simulink model "trabalhofinal_vR2012a"  (R2012a)
settings: Solver=FixedStepDiscrete  StartTime=0.0  StopTime=0.5  FixedStep=0.1e-6  MaxStep=50e-6
undefined symbols (not defined in the file): DiscIntNeverNeededParam, Ipac0, Vpac0
libraries: powerlib x36, simulink x19, fuzblock x7, powerlib_extras x2, powerlib_meascontrol x2
(part 1 of 3)
settings Model: Creator=Arthur  LastModifiedBy=Thainan
settings DataIOCC: FinalStateName=SimState  InitialState=SimState  LimitDataPoints=on  SaveCompleteFinalSimState=on  SaveFormat=Array  SignalLoggingSaveFormat=ModelDataLogs  SaveOutput=off  SignalLogging=off  DSMLogging=off  SaveTime=off  ReturnWorkspaceOutputs=off  ReturnWorkspaceOutputsName=States
settings OptimizationCC: ExpressionDepthLimit=2147483647  LifeSpan=inf  SimCompilerOptimization=Off
settings DebuggingCC: UnderspecifiedInitializationDetection=Classic  MergeDetectMultiDrivingBlocksExec=none  SolverPrmCheckMsg=warning  FcnCallInpInsideContextMsg=Enable All  StateNameClashWarn=warning  SFUnexpectedBacktrackingDiag=warning  SFNoUnconditionalDefaultTransitionDiag=warning
settings HardwareCC: ProdBitPerPointer=32  ProdLargestAtomicFloat=None  ProdIntDivRoundTo=Undefined  ProdEndianess=Unspecified  ProdWordSize=32  ProdHWDeviceType=32-bit Generic
settings ModelReferenceCC: PropagateSignalLabelsOutOfModel=off
settings SFSimCC: SimUseLocalCustomCode=off
settings RTWCC: RTWUseLocalCustomCode=off  RTWCompilerOptimization=Off
settings GRTTargetCC: CodeReplacementLibrary=C89/C90 (ANSI)  GeneratePreprocessorConditionals=Disable all  CPPClassGenCompliant=off

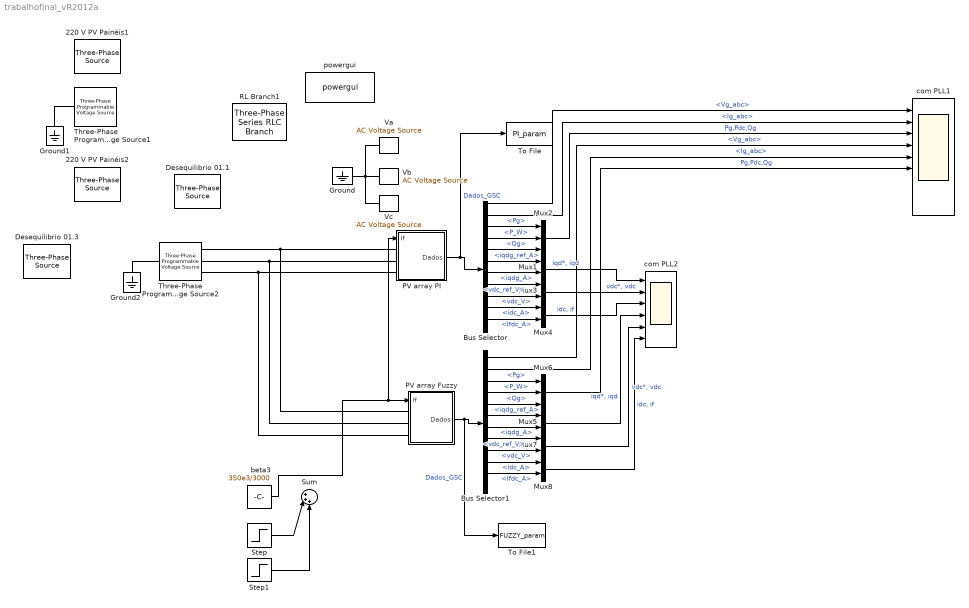
== system trabalhofinal_vR2012a ==
  220 V PV Painéis1 : powerlib/Electrical Sources/Three-Phase Source  InternalConnection=Yg  VoltagePhases=on  Voltage=120e3  PhaseAngle=0  Voltage_phases=[ 1.04183 1.09667 1.03168]*127.017  PhaseAngles_phases=[ -0.131766 -117.596 121.449]  Frequency=60  NonIdealSource=off  SpecifyImpedance=on  Resistance=0.8929  Inductance=16.58e-3  ShortCircuitLevel=100e6  BaseVoltage=120e3  XRratio=10  BusType=swing  Pref=0  Qref=0  Prefabc=[1 1 1]*400e3  Qrefabc=[1 1 1]*100  Qmin=[-1 -1 -1]*(-inf)  Qmax=[1 1 1]*inf
  220 V PV Painéis2 : powerlib/Electrical Sources/Three-Phase Source  InternalConnection=Yg  VoltagePhases=on  Voltage=120e3  PhaseAngle=0  Voltage_phases=[1 1 1]*127  PhaseAngles_phases=[ 0 -120 120]  Frequency=60  NonIdealSource=off  SpecifyImpedance=on  Resistance=0.8929  Inductance=16.58e-3  ShortCircuitLevel=100e6  BaseVoltage=120e3  XRratio=10  BusType=PQ  Pref=0  Qref=0  Prefabc=[1 1 1]*400e3  Qrefabc=[1 1 1]*100  Qmin=[-1 -1 -1]*(-inf)  Qmax=[1 1 1]*inf
  Bus Selector : BusSelector  OutputSignals=Dados_grid.Vg_abc,Dados_grid.Ig_abc,Dados_grid.Pg,DadosCC.P_W,Dados_grid.Qg,DadosCtrlCorr.iqdg_ref_A,DadosCtrlCorr.iqdg_A,DadosCtrlTensao.vdc_ref_V,DadosCtrlTensao.vdc_V,DadosCC.idc_A,DadosCC.Ifdc_A,DadosPLL.rog_rad
  Bus Selector1 : BusSelector  OutputSignals=Dados_grid.Vg_abc,Dados_grid.Ig_abc,Dados_grid.Pg,DadosCC.P_W,Dados_grid.Qg,DadosCtrlCorr.iqdg_ref_A,DadosCtrlCorr.iqdg_A,DadosCtrlTensao.vdc_ref_V,DadosCtrlTensao.vdc_V,DadosCC.idc_A,DadosCC.Ifdc_A,DadosPLL.rog_rad
  Desequilibrio 01.1 : powerlib/Electrical Sources/Three-Phase Source  InternalConnection=Yg  VoltagePhases=on  Voltage=120e3  PhaseAngle=0  Voltage_phases=[ 1.2 1 0.80]*127  PhaseAngles_phases=[ 0 -125 115]  Frequency=60  NonIdealSource=off  SpecifyImpedance=on  Resistance=0.8929  Inductance=16.58e-3  ShortCircuitLevel=100e6  BaseVoltage=120e3  XRratio=10  BusType=PQ  Pref=0  Qref=0  Prefabc=[1 1 1]*400e3  Qrefabc=[1 1 1]*100  Qmin=[-1 -1 -1]*(-inf)  Qmax=[1 1 1]*inf
  Desequilibrio 01.3 : powerlib/Electrical Sources/Three-Phase Source  InternalConnection=Yg  VoltagePhases=on  Voltage=120e3  PhaseAngle=0  Voltage_phases=[1 1 1]*440/sqrt(3)  PhaseAngles_phases=[ 0 -120 120]-90  Frequency=60  NonIdealSource=off  SpecifyImpedance=on  Resistance=0.8929  Inductance=16.58e-3  ShortCircuitLevel=100e6  BaseVoltage=120e3  XRratio=10  BusType=PQ  Pref=0  Qref=0  Prefabc=[1 1 1]*400e3  Qrefabc=[1 1 1]*100  Qmin=[-1 -1 -1]*(-inf)  Qmax=[1 1 1]*inf
  Ground : powerlib/Elements/Ground  LConnTagsString=a
  Ground1 : powerlib/Elements/Ground  LConnTagsString=a
  Ground2 : powerlib/Elements/Ground  LConnTagsString=a
  Mux{1,3..5,7..8} (6 alike) : Mux  Inputs=2
  Mux2 : Mux  Inputs=3
  Mux6 : Mux  Inputs=3
  PV array Fuzzy : Subsystem  mask(Usina Fotovoltáica){nom=[450e3 440 60], S0_pu=(350e3 +1j*0)/450e3, V0_pu=1+0*1j, C_DClink=2*4700e-6, Vdc_nom=3000, filtro_RL_pu=[0.03 0.3], GSC_PLL=[2*pi*100 sqrt(2) 2*pi*60], GSC_Ci_Ti=1e-3, GSC_Cv=[sqrt(2)  0.01*(1/1e-3)*2*pi], PWM_freq_grid=10e3, Ts_control=100e-6}
      mask prompts: nom "[Pn (VA), Vn (Vrms), fn (Hz)]:"; S0_pu "Potência aparente inicial (complexo), S0 [pu]"; V0_pu "Tensão inicial na barra (complexo), V0 [pu]"; C_DClink "C_DClink (F):"; Vdc_nom "V_DClink (V):"; filtro_RL_pu "Filtro RL [Rg_pu Lg_pu]"; GSC_PLL "Parâmetros PLL [wc qsi wff]"; GSC_Ci_Ti "Constante de tempo - Compensador de corrente GSC_Ci_Ti (s)"; GSC_Cv "Parametros controlador de tensão GSC [Cv_qsi Cv_wn]"; PWM_freq_grid "Frequencia de chaveamento do GSC"; Ts_control "Ts do controle"
      mask help: Usina fotovoltáica com inicialização.
      mask init:
      | fuzzyControl = readfis('fuzzyControl');
      | 
      | %Aquisição de dados
      | 
      | Sb = nom(1);
      | Vb = nom(2)/sqrt(3);
      | fb = nom(3); wb = 2*pi*fb;
      | S0_pu = S0_pu;
      | V0_pu = V0_pu;
      | 
      | C_DClink = C_DClink;
      | Vdc_nom = Vdc_nom;
      | 
      | Rg_pu = filtro_RL_pu(1);
      | Lg_pu = filtro_RL_pu(2);
      | 
      | GSC_PLL_wc = GSC_PLL(1);
      | GSC_PLL_qsi = GSC_PLL(2);
      | GSC_PLL_wff = GSC_PLL(3);
      | 
      | GSC_Ci_Ti = GSC_Ci_Ti;
      | 
      | GSC_Cv_qsi = GSC_Cv(1);
      | GSC_Cv_wn = GSC_Cv(2);
      | 
      | PWM_freq_grid = PWM_freq_grid;
      | 
      | Ib = Sb/(3*Vb);         % A
      | Zb = Vb/Ib;             % ohm
      | Lb = Zb/(2*pi*fb);      % Hz
      | wb = 2*pi*fb;           % rad/s
      | Yb = Vb/wb;             % wb
      | 
      | %% Condições iniciais
      | P0 = Sb*real(S0_pu);
      | Q0 = Sb*imag(S0_pu);
      | 
      | %% Controle GSC
      | % Projeto Controle de Corrente
      | Rg = Rg_pu*Zb;
      | Lg = Lg_pu*Lb;
      | 
      | GSC_Ci_kp = Lg/GSC_Ci_Ti;
      | GSC_Ci_ki = Rg/GSC_Ci_Ti;
      | 
      | %% Controle do Link DC
      | GSC_Cv_kv = -(3/2)*Vb*sqrt(2)/(Vdc_nom*C_DClink);
      | % Livro
      | 
      | GSC_Cv_kp = abs(2*GSC_Cv_qsi*GSC_Cv_wn/GSC_Cv_kv);
      | GSC_Cv_ki = abs((GSC_Cv_wn^2)/GSC_Cv_kv);
      | % Fontes Alternativas
      | % GSC_Cv_kp = 2*GSC_Cv_qsi*C_DClink*GSC_Cv_wn;
      | % GSC_Cv_ki = C_DClink*GSC_Cv_wn^2;
      | % 
      | % GSC_Cv_kp = 2.4806;
      | % GSC_Cv_ki = 667.9748;
      | 
      | %% Inicialização do Controle
      | Vgq_e = Vb*abs(V0_pu)*sqrt(2);
      | Vgd_e = 0; % PLL responsável
      | 
      | Igd_e = (2/3)*Q0/Vgq_e;
      | Igq_e = (2/3)*P0/Vgq_e;
      | 
      | GSC_Uq_e = Rg*Igq_e;
      | GSC_Ud_e = Rg*Igd_e;
      | 
      | %% Inicialização da fonte de corrente
      | If0 = P0/Vdc_nom;
      | 
      | % %% Incerteza nos parâmteros
      | % Rg = 0.8*Rg_pu*Zb;
      | % Lg = 0.8*Lg_pu*Lb;
      mask Help:
      | Dicas
      | Parâmtros da malha de corrente:
      | 	tau_i: constante de tempo de corrente 0.5 a 3ms;
      | 
      | Parâmetros do controlador de tensão
      | 	qsi_i: amortecimento critico, sqrt(2);
      | 	wn: frequência de oscilação natural.
      | 	Deve ser menor que a frequencia da malha de corrente, assim wn = 0.1*(2*pi/tau_i)]
      | 
      | Frequência de chaveamento
      | 	O valor ótimo é 10e3 Hz
      | 
      | Ts o controle
      | 	O controle pode ser feito em uma taxa de amostragem diferente da simulação do sistema, mas deve ser levado em condideração a frequência de chaveamento.
  PV array PI : Subsystem  mask(Usina Fotovoltáica){nom=[450e3 440 60], S0_pu=(350e3 +1j*0)/450e3, V0_pu=1+0*1j, C_DClink=2*4700e-6, Vdc_nom=3000, filtro_RL_pu=[0.03 0.3], GSC_PLL=[2*pi*100 sqrt(2) 2*pi*60], GSC_Ci_Ti=1e-3, GSC_Cv=[sqrt(2)  0.01*(1/1e-3)*2*pi], PWM_freq_grid=10e3, Ts_control=100e-6}
      mask prompts: nom "[Pn (VA), Vn (Vrms), fn (Hz)]:"; S0_pu "Potência aparente inicial (complexo), S0 [pu]"; V0_pu "Tensão inicial na barra (complexo), V0 [pu]"; C_DClink "C_DClink (F):"; Vdc_nom "V_DClink (V):"; filtro_RL_pu "Filtro RL [Rg_pu Lg_pu]"; GSC_PLL "Parâmetros PLL [wc qsi wff]"; GSC_Ci_Ti "Constante de tempo - Compensador de corrente GSC_Ci_Ti (s)"; GSC_Cv "Parametros controlador de tensão GSC [Cv_qsi Cv_wn]"; PWM_freq_grid "Frequencia de chaveamento do GSC"; Ts_control "Ts do controle"
      mask help: Usina fotovoltáica com inicialização.
      mask init:
      | %Aquisição de dados
      | 
      | Sb = nom(1);
      | Vb = nom(2)/sqrt(3);
      | fb = nom(3); wb = 2*pi*fb;
      | S0_pu = S0_pu;
      | V0_pu = V0_pu;
      | 
      | C_DClink = C_DClink;
      | Vdc_nom = Vdc_nom;
      | 
      | Rg_pu = filtro_RL_pu(1);
      | Lg_pu = filtro_RL_pu(2);
      | 
      | GSC_PLL_wc = GSC_PLL(1);
      | GSC_PLL_qsi = GSC_PLL(2);
      | GSC_PLL_wff = GSC_PLL(3);
      | 
      | GSC_Ci_Ti = GSC_Ci_Ti;
      | 
      | GSC_Cv_qsi = GSC_Cv(1);
      | GSC_Cv_wn = GSC_Cv(2);
      | 
      | PWM_freq_grid = PWM_freq_grid;
      | 
      | Ib = Sb/(3*Vb);         % A
      | Zb = Vb/Ib;             % ohm
      | Lb = Zb/(2*pi*fb);      % Hz
      | wb = 2*pi*fb;           % rad/s
      | Yb = Vb/wb;             % wb
      | 
      | %% Condições iniciais
      | P0 = Sb*real(S0_pu);
      | Q0 = Sb*imag(S0_pu);
      | 
      | %% Controle GSC
      | % Projeto Controle de Corrente
      | Rg = Rg_pu*Zb;
      | Lg = Lg_pu*Lb;
      | 
      | GSC_Ci_kp = (Lg)/GSC_Ci_Ti;
      | GSC_Ci_ki = (Rg)/GSC_Ci_Ti;
      | 
      | %% Controle do Link DC
      | GSC_Cv_kv = -(3/2)*Vb*sqrt(2)/(Vdc_nom*C_DClink);
      | % Livro
      | 
      | GSC_Cv_kp = abs(2*GSC_Cv_qsi*GSC_Cv_wn/GSC_Cv_kv);
      | GSC_Cv_ki = abs((GSC_Cv_wn^2)/GSC_Cv_kv);
      | % Fontes Alternativas
      | % GSC_Cv_kp = 2*GSC_Cv_qsi*C_DClink*GSC_Cv_wn;
      | % GSC_Cv_ki = C_DClink*GSC_Cv_wn^2;
      | % 
      | % GSC_Cv_kp = 2.4806;
      | % GSC_Cv_ki = 667.9748;
      | 
      | %% Inicialização do Controle
      | Vgq_e = Vb*abs(V0_pu)*sqrt(2);
      | Vgd_e = 0; % PLL responsável
      | 
      | Igd_e = (2/3)*Q0/Vgq_e;
      | Igq_e = (2/3)*P0/Vgq_e;
      | 
      | GSC_Uq_e = Rg*Igq_e;
      | GSC_Ud_e = Rg*Igd_e;
      | 
      | %% Inicialização da fonte de corrente
      | If0 = P0/Vdc_nom;
      | 
      | % %% Incerteza nos parâmteros
      | % Rg = 0.8*Rg_pu*Zb;
      | % Lg = 0.8*Lg_pu*Lb;
      mask Help:
      | Dicas
      | Parâmtros da malha de corrente:
      | 	tau_i: constante de tempo de corrente 0.5 a 3ms;
      | 
      | Parâmetros do controlador de tensão
      | 	qsi_i: amortecimento critico, sqrt(2);
      | 	wn: frequência de oscilação natural.
      | 	Deve ser menor que a frequencia da malha de corrente, assim wn = 0.1*(2*pi/tau_i)]
      | 
      | Frequência de chaveamento
      | 	O valor ótimo é 10e3 Hz
      | 
      | Ts o controle
      | 	O controle pode ser feito em uma taxa de amostragem diferente da simulação do sistema, mas deve ser levado em condideração a frequência de chaveamento.
  RL Branch1 : powerlib/Elements/Three-Phase Series RLC Branch  LConnTagsString=A|B|C  RConnTagsString=A|B|C  BranchType=RL  Resistance=0.001  Inductance=0.3e-3  Capacitance=1e-6  Measurements=None
  Step : Step  Time=0.1  After=-0.2*350e3/3000
  Step1 : Step  Time=0.25  After=0.4*350e3/3000
  Sum : Sum  Inputs=|+++
  Three-Phase Programmable Voltage Source1 : powerlib/Electrical Sources/Three-Phase Programmable Voltage Source  PositiveSequence=[220 0 60]  VariationEntity=None  VariationType=Table of time-amplitude pairs  VariationTypeAlt=Step  VariationStep=0.5  VariationRate=10  VariationMagnitude=0.3  VariationFrequency=2  VariationTiming=[1 2]  VariationPhaseA=off  Amplitudes=[1 0.5 0.5 0.5]  TimeValues=[0 0.2 0.2+5*(1/60) 2.5]  HarmonicGeneration=on  HarmonicA=[3 0.1 -25 1]  HarmonicB=[2 0.1 35 2]  Timing="[0.03  0.1]"  BusType=swing  Pref=0  Qref=0  Qmin=-inf  Qmax=inf
  Three-Phase Programmable Voltage Source2 : powerlib/Electrical Sources/Three-Phase Programmable Voltage Source  PositiveSequence=[440 -90 60]  VariationEntity=None  VariationType=Table of time-amplitude pairs  VariationTypeAlt=Step  VariationStep=0.5  VariationRate=10  VariationMagnitude=0.3  VariationFrequency=2  VariationTiming=[0.1 0.3]  VariationPhaseA=off  Amplitudes=[1 0.5 1 1]  TimeValues=[0 0.1 0.3 2.5]  HarmonicGeneration=on  HarmonicA=[3 0.1 -25 0]  HarmonicB=[2 0.2 35 2]  Timing="[0.15  0.25]"  BusType=swing  Pref=0  Qref=0  Qmin=-inf  Qmax=inf
  To File : ToFile  Filename=PI_param  MatrixName=PI  SaveFormat=Timeseries
  To File1 : ToFile  Filename=FUZZY_param  MatrixName=FUZZY  SaveFormat=Timeseries
  Va : powerlib/Electrical Sources/AC Voltage Source  Amplitude=180  Phase=0  Frequency=60  SampleTime=0  Measurements=None  BusType=swing  Pref=10e3  Qref=0  Qmin=-inf  Qmax=+inf
  Vb : powerlib/Electrical Sources/AC Voltage Source  Amplitude=180  Phase=-120  Frequency=60  SampleTime=0  Measurements=None  BusType=swing  Pref=10e3  Qref=0  Qmin=-inf  Qmax=+inf
  Vc : powerlib/Electrical Sources/AC Voltage Source  Amplitude=180  Phase=120  Frequency=60  SampleTime=0  Measurements=None  BusType=swing  Pref=10e3  Qref=0  Qmin=-inf  Qmax=+inf
  beta3 : Constant  Value=350e3/3000  SampleTime=-1
  com PLL1 : Scope  NumInputPorts=9
      settings: TimeRange=0.1  MaxDataPoints=5000  SaveToWorkspace=off  SaveName=ScopeData3  YMin=-479.80883~-996.40535~-2695635.97068~-479.80883~-1014.51596~-2755857.55084~-1.00000~-1.00000~-116.66666666666681  YMax=515.48883~956.94474~763486.7953~515.48883~965.23302~776717.6903~1.00000~1.00000~-116.66666666666666  SampleTime=-1
  com PLL2 : Scope  NumInputPorts=6
      settings: TimeRange=0.1  MaxDataPoints=5000  SaveToWorkspace=off  SaveName=ScopeData2  YMin=-218.09144~2992.71371~-879.19718~-220.1817~2995.0846~-898.81456  YMax=911.90416~3017.07049~98.28703~930.71651~3018.04175~100.46674  SampleTime=-1
  powergui : powerlib/powergui  Priority=1  SimulationMode=Discrete  SolverType=Tustin  SampleTime=0.1e-6  frequency=60  SPID=off  DisableSnubberDevices=off  DisableRonSwitches=off  DisableVfSwitches=off  SwTol=0  DisplayEquations=off  Interpol=off  ExternalGateDelay=off  methode=off  Ts=0  FunctionMessages=off  echomessages=off  HookPort=off  EnableUseOfTLC=off  x0status=blocks  frequencyindice=0  Pbase=100e6  ErrMax=1e-4  Iterations=50  UnitsV=kV  UnitsW=MW  buscounter=0  RestoreLinks=warning  ResistiveCurrentMeasurement=off  Frange=[0:2:500]  Ylog=off  Xlog=on  ShowGrid=off  save=off  variable=ZData  structure=0  ZoomFFT=off  StartTime=0.0  cycles=1  DisplayStyle=1  fundamental=60  FreqAxis=off  MaxFrequency=1000  frequencyindicesteady=1  RmsSteady=1  display=off
  wires:
  PV array PI/1(Dados) -> To File/1, Bus Selector/1  "Dados_GSC"
  Bus Selector/1 -> com PLL1/1  "<Vg_abc>"
  Bus Selector/2 -> com PLL1/2  "<Ig_abc>"
  Bus Selector/3 -> Mux2/1  "<Pg>"
  Bus Selector/5 -> Mux2/3  "<Qg>"
  Mux2/1 -> com PLL1/3  "Pg,Pdc,Qg"
  Bus Selector/6 -> Mux1/1  "<iqdg_ref_A>"
  Bus Selector/7 -> Mux1/2  "<iqdg_A>"
  Bus Selector/8 -> Mux3/1  "<vdc_ref_V>"
  Bus Selector/9 -> Mux3/2  "<vdc_V>"
  Mux1/1 -> com PLL2/1  "iqd*, iqd"
  Mux3/1 -> com PLL2/2  "vdc*, vdc"
  Bus Selector/10 -> Mux4/1  "<idc_A>"
  Bus Selector/4 -> Mux2/2  "<P_W>"
  Bus Selector/11 -> Mux4/2  "<Ifdc_A>"
  Mux4/1 -> com PLL2/3  "idc, if"
  PV array Fuzzy/1(Dados) -> To File1/1, Bus Selector1/1  "Dados_GSC"
  Bus Selector1/1 -> com PLL1/4  "<Vg_abc>"
  Bus Selector1/2 -> com PLL1/5  "<Ig_abc>"
  Bus Selector1/3 -> Mux6/1  "<Pg>"
  Bus Selector1/5 -> Mux6/3  "<Qg>"
  Mux6/1 -> com PLL1/6  "Pg,Pdc,Qg"
  Bus Selector1/6 -> Mux5/1  "<iqdg_ref_A>"
  Bus Selector1/7 -> Mux5/2  "<iqdg_A>"
  Bus Selector1/8 -> Mux7/1  "<vdc_ref_V>"
  Bus Selector1/9 -> Mux7/2  "<vdc_V>"
  Mux5/1 -> com PLL2/4  "iqd*, iqd"
  Mux7/1 -> com PLL2/5  "vdc*, vdc"
  Bus Selector1/10 -> Mux8/1  "<idc_A>"
  Bus Selector1/4 -> Mux6/2  "<P_W>"
  Bus Selector1/11 -> Mux8/2  "<Ifdc_A>"
  Mux8/1 -> com PLL2/6  "idc, if"
  Step/1 -> Sum/2
  Step1/1 -> Sum/3
  beta3/1 -> PV array PI/1(If), PV array Fuzzy/1(If)
  connections:
  Three-Phase Programmable Voltage Source2/RConn2 -- PV array Fuzzy/LConn2 -- PV array PI/LConn2
  Three-Phase Programmable Voltage Source2/RConn1 -- PV array Fuzzy/LConn1 -- PV array PI/LConn1
  Ground1/LConn1 -- Three-Phase Programmable Voltage Source1/LConn1
  Ground/LConn1 -- Vc/LConn1 -- Va/LConn1 -- Vb/LConn1
  Three-Phase Programmable Voltage Source2/RConn3 -- PV array Fuzzy/LConn3 -- PV array PI/LConn3
  Ground2/LConn1 -- Three-Phase Programmable Voltage Source2/LConn1

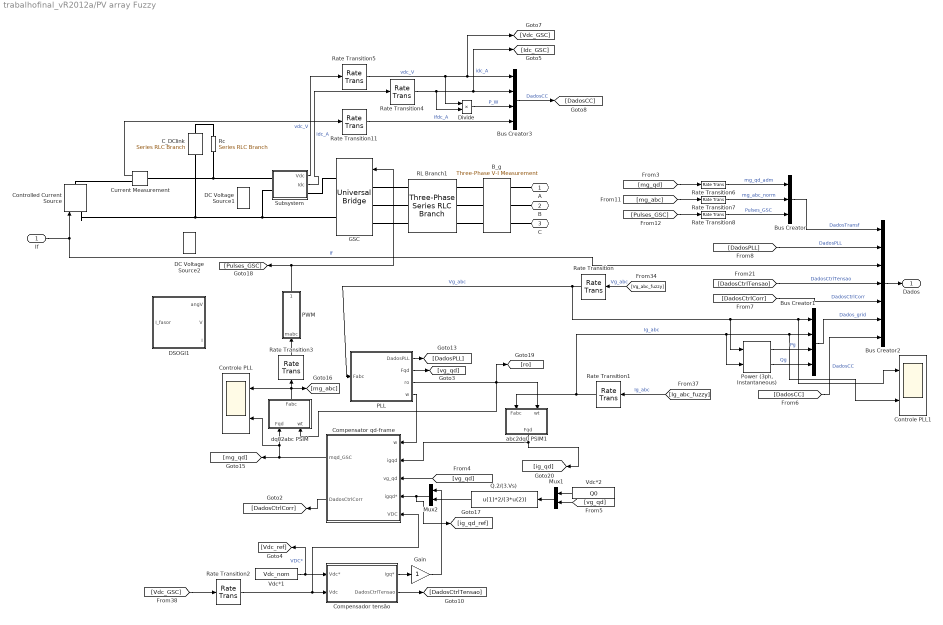
== system trabalhofinal_vR2012a/PV array Fuzzy ==
  If : Inport
  B_g : powerlib/Measurements/Three-Phase V-I Measurement  VoltageMeasurement=phase-to-ground  SetLabelV=on  LabelV=Vg_abc_fuzzy  Vpu=off  VpuLL=off  CurrentMeasurement=yes  SetLabelI=on  LabelI=Ig_abc_fuzzy  Ipu=off  Pbase=Pnom  Vbase=0  OutputType=Complex  PhasorSimulation=off  PSBequivalent=0
  Bus Creator : BusCreator  Inputs=3
  Bus Creator1 : BusCreator  Inputs=4
  Bus Creator2 : BusCreator  Inputs=7
  Bus Creator3 : BusCreator  Inputs=4
  C_DClink : powerlib/Elements/Series RLC Branch  LConnTagsString=__new0  RConnTagsString=__new0  BranchType=C  Resistance=1  Inductance=1e-3  SetiL0=off  InitialCurrent=0  Capacitance=C_DClink  Setx0=on  InitialVoltage=Vdc_nom  Measurements=None
  Compensador tensão : Subsystem
  Compensator qd-frame : Subsystem
  Controle PLL : Scope  NumInputPorts=2
      settings: TimeRange=auto  MaxDataPoints=5000  SaveToWorkspace=off  SaveName=ScopeData6  YMin=-1.09366~-0.29006  YMax=1.05813~1.00993  SampleTime=-1
  Controle PLL1 : Scope  NumInputPorts=2
      settings: TimeRange=auto  ShowLegends=on  MaxDataPoints=5000  SaveToWorkspace=off  YMin=-959.21545~-765.38646  YMax=959.27732~778.48408  SampleTime=-1
  Controlled Current Source : powerlib/Electrical Sources/Controlled Current Source  Initialize=on  Source_Type=AC  Amplitude=If0  Phase=0  Frequency=0  Measurements=None
  Current Measurement : powerlib/Measurements/Current Measurement  PhasorSimulation=off  OutputType=Complex  PSBequivalent=0
  DC Voltage Source1 : powerlib/Electrical Sources/DC Voltage Source  Amplitude=Vdc_nom  Measurements=None
  DC Voltage Source2 : powerlib/Electrical Sources/DC Voltage Source  Amplitude=Vdc_nom  Measurements=None
  DSOGI1 : Subsystem  mask{Vp=sqrt(2)*abs(Vpac0), wc_PLL=2*pi*100, wB=2*pi*60, qsi_PLL=sqrt(2), v0_fasor=Vpac0*exp(-1j*pi/2), i0_fasor=Ipac0*exp(-1j*pi/2)}
      mask prompts: Vp "Valor de pico da tensão, Vp"; wc_PLL "Frequencia de corte PLL, wc_PLL [rad/s]"; wB "Frequência basel, wB [rad]"; qsi_PLL "Fator de amortecimento PLL, qsi_PLL"; v0_fasor "Fasor Inicial de tensão, v0_fasor [pu]"; i0_fasor "Fasor Inicial de corrente, i0_fasor [pu]"
      mask init:
      | % Ganhos do compensador PLL
      | kp_PLL = 2*qsi_PLL*wc_PLL;
      | ki_PLL = wc_PLL^2;
      | k = sqrt(2);
      | 
      | % Valores Iniciais: alfa/beta
      | val0 = sqrt(2)*real(v0_fasor);
      | vbe0 = sqrt(2)*imag(v0_fasor);
      | ial0 = sqrt(2)*real(i0_fasor);
      | ibe0 = sqrt(2)*imag(i0_fasor);
      | 
      | phase0_v = phase(v0_fasor);
      | 
      | % Valores linha
      | val0_lin = (1/2)*val0; % int1
      | vbe0_lin = (1/2)*vbe0; % int3
      | 
      | ial0_lin = (1/2)*ial0; 
      | ibe0_lin = (1/2)*ibe0;
      | 
      | % Valores quadratura linha
      | qval0_lin = vbe0_lin; % int2
      | qvbe0_lin = -val0_lin; % int4
      | 
      | qial0_lin = ibe0_lin;
      | qibe0_lin = -ial0_lin;
      | 
      | 
      | 
      | int1_v = val0_lin;
      | int2_v = qval0_lin;
      | int3_v = vbe0_lin;
      | int4_v = qvbe0_lin;
      | 
      | int1_i = ial0_lin;
      | int2_i = qial0_lin;
      | int3_i = ibe0_lin;
      | int4_i = qibe0_lin;
  Divide : Product  Inputs=**
  GSC : powerlib/Power Electronics/Universal Bridge  Arms=3  SnubberResistance=1e5  SnubberCapacitance=inf  Device=IGBT / Diodes  Ron=1e-3  Lon=0  ForwardVoltages="[  0  0  ]"  ForwardVoltage=0  GTOparameters=[ 10e-6 , 20e-6 ]  IGBTparameters=[ 1e-6 , 2e-6 ]  Measurements=None  Measurements_2=None  converterType=Rectifier
  Gain : Gain
  Mux1 : Mux  Inputs=2
  Mux2 : Mux  Inputs=2
  PLL : Subsystem  mask{Fp=abs(Vb*V0_pu)*sqrt(2), Ci=[GSC_PLL_wc GSC_PLL_qsi], wff=GSC_PLL_wff, v0_pu=V0_pu}
      mask prompts: Fp "Valor de pico, Fp"; Ci "Compensador, [wc qsi]"; wff "Frequência central, wff [rad/s]"; v0_pu "Condições Iniciais fasor v0_pu"
      mask init:
      | wc = Ci(1);
      | qsi = Ci(2);
      | kp = 2*qsi*wc;
      | ki = wc^2;
      | dw0 = 0;
      | ro0 = (phase(v0_pu)-pi/2);
  PWM : Subsystem
  "Power (3ph, Instantaneous)" : powerlib_meascontrol/Measurements/Power (3ph, Instantaneous)
  Q.2/(3.Vs) : Fcn  Expr=u(1)*2/(3*u(2))
  RL Branch1 : powerlib/Elements/Three-Phase Series RLC Branch  LConnTagsString=A|B|C  RConnTagsString=A|B|C  BranchType=RL  Resistance=Rg  Inductance=Lg  Capacitance=1e-6  Measurements=None
  Rate Transition{,1..2,4..8,11} (9 alike) : RateTransition  OutPortSampleTime=Ts_control
  Rate Transition3 : RateTransition
  Rc : powerlib/Elements/Series RLC Branch  LConnTagsString=__new0  RConnTagsString=__new0  BranchType=R  Resistance=1e-6  Inductance=450e-3  SetiL0=on  InitialCurrent=0  Capacitance=0  Setx0=off  InitialVoltage=0  Measurements=None
  Subsystem : Subsystem
  Vdc*1 : Constant  Value=Vdc_nom  SampleTime=-1
  Vdc*2 : Constant  Value=Q0  SampleTime=-1
  abc2dq0 PSIM1 : Subsystem
  dq02abc PSIM : Subsystem
  A : PMIOPort  Port=1  Side=Left
  B : PMIOPort  Port=2  Side=Left
  C : PMIOPort  Port=3  Side=Left
  Dados : Outport
  wires:
  PWM/1(Pulses) -> GSC/1, [Pulses_GSC]
  Subsystem/1(Vdc) -> Rate Transition5/1  "vdc_V"
  Compensador tensão/1(igq*) -> Gain/1
  Bus Creator2/1 -> Dados/1
  abc2dq0 PSIM1/1(Fqd) -> Compensator qd-frame/2(igqd), [ig_qd]
  [vg_qd] -> Compensator qd-frame/3(vg_qd)
  Vdc*1/1 -> Compensador tensão/1(Vdc*), [Vdc_ref]  "VDC*"
  Compensator qd-frame/1(mqd_GSC) -> Controle PLL/2, dq02abc PSIM/1(Fqd), [mg_qd]
  [mg_qd] -> Rate Transition6/1
  [mg_abc] -> Rate Transition7/1
  [Pulses_GSC] -> Rate Transition8/1
  [Vdc_GSC] -> Rate Transition2/1
  Compensador tensão/2(DadosCtrlTensao) -> [DadosCtrlTensao]
  Compensator qd-frame/2(DadosCtrlCorr) -> [DadosCtrlCorr]
  [DadosCtrlTensao] -> Bus Creator2/4  "DadosCtrlTensao"
  [DadosCtrlCorr] -> Bus Creator2/5  "DadosCtrlCorr"
  [DadosPLL] -> Bus Creator2/2  "DadosPLL"
  Bus Creator/1 -> Bus Creator2/1  "DadosTransf"
  dq02abc PSIM/1(Fabc) -> [mg_abc], Controle PLL/1, Rate Transition3/1
  Mux2/1 -> Compensator qd-frame/4(igqd*), [ig_qd_ref]
  Q.2/(3.Vs)/1 -> Mux2/2
  Gain/1 -> Mux2/1
  [Ig_abc_fuzzy] -> Rate Transition1/1  "Ig_abc"
  "Power (3ph, Instantaneous)"/2 -> Bus Creator1/4  "Qg"
  "Power (3ph, Instantaneous)"/1 -> Bus Creator1/3  "Pg"
  Bus Creator1/1 -> Bus Creator2/6  "Dados_grid"
  If/1 -> Controlled Current Source/1, Bus Creator2/3  "If"
  Rate Transition2/1 -> Compensator qd-frame/5(VDC), Compensador tensão/2(Vdc)
  Rate Transition3/1 -> PWM/1(mabc)
  PLL/1(DadosPLL) -> [DadosPLL]
  PLL/2(Fqd) -> [vg_qd]
  PLL/3(ro) -> dq02abc PSIM/2(wt), abc2dq0 PSIM1/2(wt), [ro]
  Subsystem/2(Idc) -> Rate Transition4/1  "idc_A"
  Divide/1 -> Bus Creator3/3  "P_W"
  Bus Creator3/1 -> [DadosCC]  "DadosCC"
  [DadosCC] -> Bus Creator2/7  "DadosCC"
  Rate Transition4/1 -> Divide/2, Bus Creator3/2, [Idc_GSC]  "idc_A"
  Rate Transition5/1 -> [Vdc_GSC], Bus Creator3/1, Divide/1  "vdc_V"
  Rate Transition6/1 -> Bus Creator/1  "mg_qd_adm"
  Rate Transition7/1 -> Bus Creator/2  "mg_abc_norm"
  Rate Transition8/1 -> Bus Creator/3  "Pulses_GSC"
  Rate Transition/1 -> "Power (3ph, Instantaneous)"/1, Controle PLL1/1, Bus Creator1/1, PLL/1(Fabc)  "Vg_abc"
  Rate Transition1/1 -> "Power (3ph, Instantaneous)"/2, Controle PLL1/2, Bus Creator1/2, abc2dq0 PSIM1/1(Fabc)  "Ig_abc"
  Current Measurement/1 -> Rate Transition11/1
  Rate Transition11/1 -> Bus Creator3/4  "Ifdc_A"
  Vdc*2/1 -> Mux1/1
  [vg_qd] -> Mux1/2
  Mux1/1 -> Q.2/(3.Vs)/1
  [Vg_abc_fuzzy] -> Rate Transition/1  "Vg_abc"
  PLL/4(w) -> Compensator qd-frame/1(w)
  connections:
  B_g/RConn1 -- A/RConn1
  B_g/RConn2 -- B/RConn1
  B_g/RConn3 -- C/RConn1
  RL Branch1/LConn3 -- GSC/LConn3
  RL Branch1/LConn1 -- GSC/LConn1
  RL Branch1/LConn2 -- GSC/LConn2
  RL Branch1/RConn1 -- B_g/LConn1
  RL Branch1/RConn3 -- B_g/LConn3
  RL Branch1/RConn2 -- B_g/LConn2
  Subsystem/RConn1 -- GSC/RConn1
  Rc/LConn1 -- C_DClink/LConn1
  Current Measurement/RConn1 -- Controlled Current Source/RConn1
  Controlled Current Source/LConn1 -- C_DClink/RConn1 -- GSC/RConn2 -- Subsystem/LConn2
  Rc/RConn1 -- Subsystem/LConn1 -- Current Measurement/LConn1

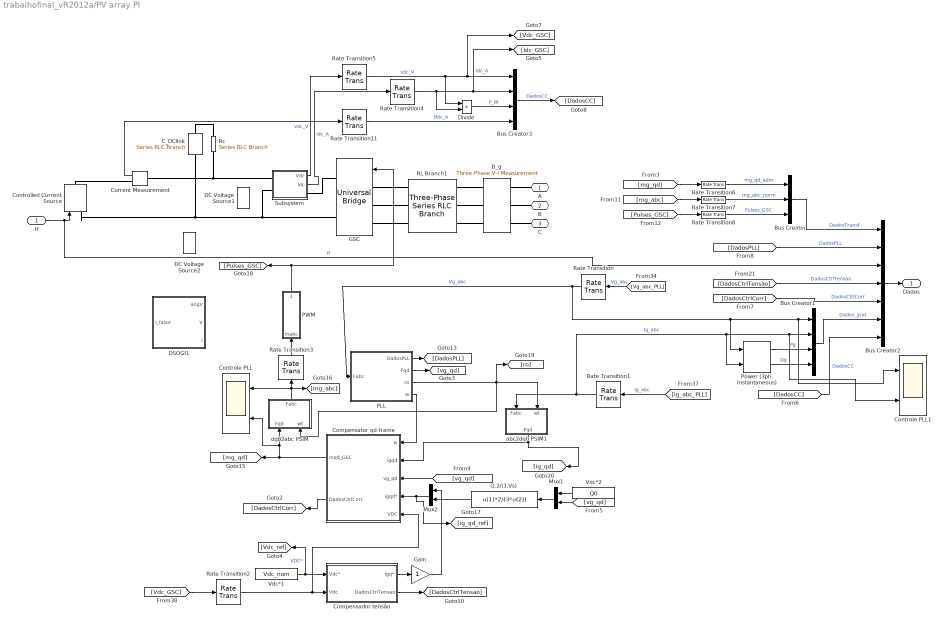
== system trabalhofinal_vR2012a/PV array PI ==
  If : Inport
  B_g : powerlib/Measurements/Three-Phase V-I Measurement  VoltageMeasurement=phase-to-ground  SetLabelV=on  LabelV=Vg_abc_PLL  Vpu=off  VpuLL=off  CurrentMeasurement=yes  SetLabelI=on  LabelI=Ig_abc_PLL  Ipu=off  Pbase=Pnom  Vbase=0  OutputType=Complex  PhasorSimulation=off  PSBequivalent=0
  Bus Creator : BusCreator  Inputs=3
  Bus Creator1 : BusCreator  Inputs=4
  Bus Creator2 : BusCreator  Inputs=7
  Bus Creator3 : BusCreator  Inputs=4
  C_DClink : powerlib/Elements/Series RLC Branch  LConnTagsString=__new0  RConnTagsString=__new0  BranchType=C  Resistance=1  Inductance=1e-3  SetiL0=off  InitialCurrent=0  Capacitance=C_DClink  Setx0=on  InitialVoltage=Vdc_nom  Measurements=None
  Compensador tensão : Subsystem
  Compensator qd-frame : Subsystem
  Controle PLL : Scope  NumInputPorts=2
      settings: TimeRange=auto  MaxDataPoints=5000  SaveToWorkspace=off  SaveName=ScopeData6  YMin=-0.67408~-0.16999  YMax=0.65921~0.69985  SampleTime=-1
  Controle PLL1 : Scope  NumInputPorts=2
      settings: TimeRange=auto  ShowLegends=on  MaxDataPoints=5000  SaveToWorkspace=off  YMin=-959.21545~-765.38646  YMax=959.27732~778.48408  SampleTime=-1
  Controlled Current Source : powerlib/Electrical Sources/Controlled Current Source  Initialize=on  Source_Type=AC  Amplitude=If0  Phase=0  Frequency=0  Measurements=None
  Current Measurement : powerlib/Measurements/Current Measurement  PhasorSimulation=off  OutputType=Complex  PSBequivalent=0
  DC Voltage Source1 : powerlib/Electrical Sources/DC Voltage Source  Amplitude=Vdc_nom  Measurements=None
  DC Voltage Source2 : powerlib/Electrical Sources/DC Voltage Source  Amplitude=Vdc_nom  Measurements=None
  DSOGI1 : Subsystem  mask{Vp=sqrt(2)*abs(Vpac0), wc_PLL=2*pi*100, wB=2*pi*60, qsi_PLL=sqrt(2), v0_fasor=Vpac0*exp(-1j*pi/2), i0_fasor=Ipac0*exp(-1j*pi/2)}
      mask prompts: Vp "Valor de pico da tensão, Vp"; wc_PLL "Frequencia de corte PLL, wc_PLL [rad/s]"; wB "Frequência basel, wB [rad]"; qsi_PLL "Fator de amortecimento PLL, qsi_PLL"; v0_fasor "Fasor Inicial de tensão, v0_fasor [pu]"; i0_fasor "Fasor Inicial de corrente, i0_fasor [pu]"
      mask init: same as trabalhofinal_vR2012a/PV array Fuzzy/DSOGI1
  Divide : Product  Inputs=**
  GSC : powerlib/Power Electronics/Universal Bridge  Arms=3  SnubberResistance=1e5  SnubberCapacitance=inf  Device=IGBT / Diodes  Ron=1e-3  Lon=0  ForwardVoltages="[  0  0  ]"  ForwardVoltage=0  GTOparameters=[ 10e-6 , 20e-6 ]  IGBTparameters=[ 1e-6 , 2e-6 ]  Measurements=None  Measurements_2=None  converterType=Rectifier
  Gain : Gain
  Mux1 : Mux  Inputs=2
  Mux2 : Mux  Inputs=2
  PLL : Subsystem  mask{Fp=abs(Vb*V0_pu)*sqrt(2), Ci=[GSC_PLL_wc GSC_PLL_qsi], wff=GSC_PLL_wff, v0_pu=V0_pu}
      mask prompts: Fp "Valor de pico, Fp"; Ci "Compensador, [wc qsi]"; wff "Frequência central, wff [rad/s]"; v0_pu "Condições Iniciais fasor v0_pu"
      mask init:
      | wc = Ci(1);
      | qsi = Ci(2);
      | kp = 2*qsi*wc;
      | ki = wc^2;
      | dw0 = 0;
      | ro0 = (phase(v0_pu)-pi/2);
  PWM : Subsystem
  "Power (3ph, Instantaneous)" : powerlib_meascontrol/Measurements/Power (3ph, Instantaneous)
  Q.2/(3.Vs) : Fcn  Expr=u(1)*2/(3*u(2))
  RL Branch1 : powerlib/Elements/Three-Phase Series RLC Branch  LConnTagsString=A|B|C  RConnTagsString=A|B|C  BranchType=RL  Resistance=Rg  Inductance=Lg  Capacitance=1e-6  Measurements=None
  Rate Transition{,1..2,4..8,11} (9 alike) : RateTransition  OutPortSampleTime=Ts_control
  Rate Transition3 : RateTransition
  Rc : powerlib/Elements/Series RLC Branch  LConnTagsString=__new0  RConnTagsString=__new0  BranchType=R  Resistance=1e-6  Inductance=450e-3  SetiL0=on  InitialCurrent=0  Capacitance=0  Setx0=off  InitialVoltage=0  Measurements=None
  Subsystem : Subsystem
  Vdc*1 : Constant  Value=Vdc_nom  SampleTime=-1
  Vdc*2 : Constant  Value=Q0  SampleTime=-1
  abc2dq0 PSIM1 : Subsystem
  dq02abc PSIM : Subsystem
  A : PMIOPort  Port=1  Side=Left
  B : PMIOPort  Port=2  Side=Left
  C : PMIOPort  Port=3  Side=Left
  Dados : Outport
  wires:
  PWM/1(Pulses) -> GSC/1, [Pulses_GSC]
  Subsystem/1(Vdc) -> Rate Transition5/1  "vdc_V"
  Compensador tensão/1(igq*) -> Gain/1
  Bus Creator2/1 -> Dados/1
  abc2dq0 PSIM1/1(Fqd) -> Compensator qd-frame/2(igqd), [ig_qd]
  [vg_qd] -> Compensator qd-frame/3(vg_qd)
  Vdc*1/1 -> Compensador tensão/1(Vdc*), [Vdc_ref]  "VDC*"
  Compensator qd-frame/1(mqd_GSC) -> Controle PLL/2, dq02abc PSIM/1(Fqd), [mg_qd]
  [mg_qd] -> Rate Transition6/1
  [mg_abc] -> Rate Transition7/1
  [Pulses_GSC] -> Rate Transition8/1
  [Vdc_GSC] -> Rate Transition2/1
  Compensador tensão/2(DadosCtrlTensao) -> [DadosCtrlTensao]
  Compensator qd-frame/2(DadosCtrlCorr) -> [DadosCtrlCorr]
  [DadosCtrlTensao] -> Bus Creator2/4  "DadosCtrlTensao"
  [DadosCtrlCorr] -> Bus Creator2/5  "DadosCtrlCorr"
  [DadosPLL] -> Bus Creator2/2  "DadosPLL"
  Bus Creator/1 -> Bus Creator2/1  "DadosTransf"
  dq02abc PSIM/1(Fabc) -> [mg_abc], Controle PLL/1, Rate Transition3/1
  Mux2/1 -> Compensator qd-frame/4(igqd*), [ig_qd_ref]
  Q.2/(3.Vs)/1 -> Mux2/2
  Gain/1 -> Mux2/1
  [Ig_abc_PLL] -> Rate Transition1/1  "Ig_abc"
  "Power (3ph, Instantaneous)"/2 -> Bus Creator1/4  "Qg"
  "Power (3ph, Instantaneous)"/1 -> Bus Creator1/3  "Pg"
  Bus Creator1/1 -> Bus Creator2/6  "Dados_grid"
  If/1 -> Bus Creator2/3, Controlled Current Source/1  "If"
  Rate Transition2/1 -> Compensator qd-frame/5(VDC), Compensador tensão/2(Vdc)
  Rate Transition3/1 -> PWM/1(mabc)
  PLL/1(DadosPLL) -> [DadosPLL]
  PLL/2(Fqd) -> [vg_qd]
  PLL/3(ro) -> dq02abc PSIM/2(wt), abc2dq0 PSIM1/2(wt), [ro]
  Subsystem/2(Idc) -> Rate Transition4/1  "idc_A"
  Divide/1 -> Bus Creator3/3  "P_W"
  Bus Creator3/1 -> [DadosCC]  "DadosCC"
  [DadosCC] -> Bus Creator2/7  "DadosCC"
  Rate Transition4/1 -> Divide/2, Bus Creator3/2, [Idc_GSC]  "idc_A"
  Rate Transition5/1 -> [Vdc_GSC], Bus Creator3/1, Divide/1  "vdc_V"
  Rate Transition6/1 -> Bus Creator/1  "mg_qd_adm"
  Rate Transition7/1 -> Bus Creator/2  "mg_abc_norm"
  Rate Transition8/1 -> Bus Creator/3  "Pulses_GSC"
  Rate Transition/1 -> "Power (3ph, Instantaneous)"/1, Controle PLL1/1, Bus Creator1/1, PLL/1(Fabc)  "Vg_abc"
  Rate Transition1/1 -> "Power (3ph, Instantaneous)"/2, Controle PLL1/2, Bus Creator1/2, abc2dq0 PSIM1/1(Fabc)  "Ig_abc"
  Current Measurement/1 -> Rate Transition11/1
  Rate Transition11/1 -> Bus Creator3/4  "Ifdc_A"
  Vdc*2/1 -> Mux1/1
  [vg_qd] -> Mux1/2
  Mux1/1 -> Q.2/(3.Vs)/1
  [Vg_abc_PLL] -> Rate Transition/1  "Vg_abc"
  PLL/4(w) -> Compensator qd-frame/1(w)
  connections:
  B_g/RConn1 -- A/RConn1
  B_g/RConn2 -- B/RConn1
  B_g/RConn3 -- C/RConn1
  RL Branch1/LConn3 -- GSC/LConn3
  RL Branch1/LConn1 -- GSC/LConn1
  RL Branch1/LConn2 -- GSC/LConn2
  RL Branch1/RConn1 -- B_g/LConn1
  RL Branch1/RConn3 -- B_g/LConn3
  RL Branch1/RConn2 -- B_g/LConn2
  Subsystem/RConn1 -- GSC/RConn1
  Rc/LConn1 -- C_DClink/LConn1
  Current Measurement/RConn1 -- Controlled Current Source/RConn1
  Controlled Current Source/LConn1 -- C_DClink/RConn1 -- GSC/RConn2 -- Subsystem/LConn2
  Rc/RConn1 -- Subsystem/LConn1 -- Current Measurement/LConn1

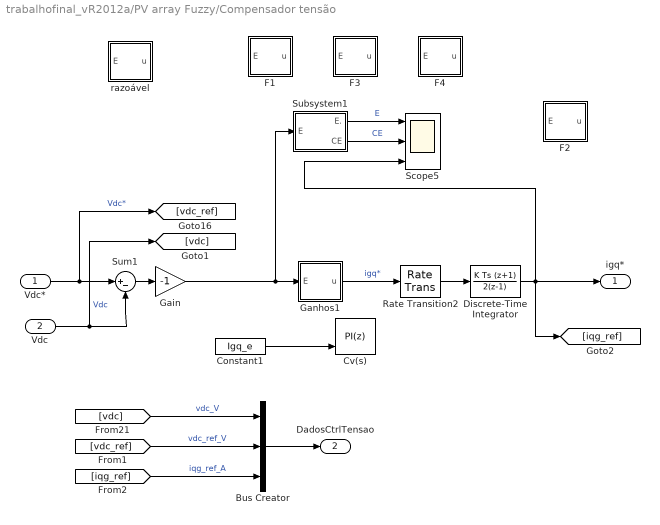
== system trabalhofinal_vR2012a/PV array Fuzzy/Compensador tensão ==
  Vdc* : Inport
  Vdc : Inport  Port=2
  Bus Creator : BusCreator  Inputs=3
  Constant1 : Constant  Value=Igq_e
  Cv(s) : simulink/Continuous/PID Controller  Controller=PI  TimeDomain=Discrete-time  SampleTime=-1  IntegratorMethod=Trapezoidal  FilterMethod=Forward Euler  Form=Parallel  UseFilter=on  ControllerParametersSource=internal  P=GSC_Cv_kp  I=GSC_Cv_ki  D=0  N=100  InitialConditionSource=external  InitialConditionForIntegrator=0  InitialConditionForFilter=0  ExternalReset=none  LimitOutput=off  UpperSaturationLimit=inf  LowerSaturationLimit=-inf  LinearizeAsGain=on  AntiWindupMode=none  Kb=1  TrackingMode=off  Kt=1  PParamMin=[]  PParamMax=[]  IParamMin=[]  IParamMax=[]  DParamMin=[]  DParamMax=[]  NParamMin=[]  NParamMax=[]  KbParamMin=[]  KbParamMax=[]  KtParamMin=[]  KtParamMax=[]  POutMin=[]  POutMax=[]  IOutMin=[]  IOutMax=[]  DOutMin=[]  DOutMax=[]  NOutMin=[]  NOutMax=[]  KbOutMin=[]  KbOutMax=[]  KtOutMin=[]  KtOutMax=[]  IntegratorOutMin=[]  IntegratorOutMax=[]  FilterOutMin=[]  FilterOutMax=[]  SumOutMin=[]  SumOutMax=[]  SumI1OutMin=[]  SumI1OutMax=[]  SumI2OutMin=[]  SumI2OutMax=[]  SumI3OutMin=[]  SumI3OutMax=[]  SumDOutMin=[]  SumDOutMax=[]  SaturationOutMin=[]  SaturationOutMax=[]  IntegratorContinuousStateAttributes=''  IntegratorStateMustResolveToSignalObject=off  IntegratorRTWStateStorageClass=Auto  FilterContinuousStateAttributes=''  FilterStateMustResolveToSignalObject=off  FilterRTWStateStorageClass=Auto  DifferentiatorICPrevScaledInput=0  DifferentiatorOutMin=[]  DifferentiatorOutMax=[]
  Discrete-Time Integrator : DiscreteIntegrator  IntegratorMethod=Integration: Trapezoidal  InitialCondition=Igq_e  InitialConditionMode=State only (most efficient)  SampleTime=-1  ICPrevOutput=DiscIntNeverNeededParam  ICPrevScaledInput=DiscIntNeverNeededParam
  F1 : Subsystem  mask{GE=100, GCE=1/50000, GY=2000, Ts_fuzzy=0.001e-3}
      mask prompts: GE "Fator erro, GE"; GCE "Fator mudança erro, GCE"; GY "Fator Saída, GY"; Ts_fuzzy "Periodo amostragem"
  F2 : Subsystem  mask{GE=300, GCE=1/300e3, GY=2e3, Ts_fuzzy=10e-6}
      mask prompts: GE "Fator erro, GE"; GCE "Fator mudança erro, GCE"; GY "Fator Saída, GY"; Ts_fuzzy "Periodo amostragem"
  F3 : Subsystem  mask{GE=1/100, GCE=1/100e4, GY=2e3, Ts_fuzzy=0.1e-3}
      mask prompts: GE "Fator erro, GE"; GCE "Fator mudança erro, GCE"; GY "Fator Saída, GY"; Ts_fuzzy "Periodo amostragem"
  F4 : Subsystem  mask{GE=1/10, GCE=1/100e4, GY=2e3, Ts_fuzzy=0.1e-3}
      mask prompts: GE "Fator erro, GE"; GCE "Fator mudança erro, GCE"; GY "Fator Saída, GY"; Ts_fuzzy "Periodo amostragem"
  Gain : Gain  Gain=-1
  Ganhos1 : Subsystem  mask{GE=1/(2*GSC_Cv_kp), GCE=1/(10*GSC_Cv_ki), GY=100*Igq_e, Ts_fuzzy=100e-6}
      mask prompts: GE "Fator erro, GE"; GCE "Fator mudança erro, GCE"; GY "Fator Saída, GY"; Ts_fuzzy "Periodo amostragem"
  Rate Transition2 : RateTransition  X0=Igq_e  OutPortSampleTime=Ts_control
  Scope5 : Scope  NumInputPorts=3
      settings: TimeRange=auto  MaxDataPoints=5000  SaveToWorkspace=off  SaveName=ScopeData4  YMin=-6.80779~-4917.32396~441.47301  YMax=15.48373~16753.67536~853.61798  SampleTime=-1
  Subsystem1 : Subsystem
  Sum1 : Sum  Inputs=|+-
  razoável : Subsystem  mask{GE=1/20, GCE=1/(5*4e4), GY=3e3}
      mask prompts: GE "Fator erro"; GCE "Fator mudança erro"; GY "Fator Saída"
  igq* : Outport
  DadosCtrlTensao : Outport  Port=2
  wires:
  Constant1/1 -> Cv(s)/2
  Vdc*/1 -> [vdc_ref], Sum1/1  "Vdc*"
  Vdc/1 -> [vdc], Sum1/2  "Vdc"
  Sum1/1 -> Gain/1
  [vdc] -> Bus Creator/1  "vdc_V"
  [vdc_ref] -> Bus Creator/2  "vdc_ref_V"
  [iqg_ref] -> Bus Creator/3  "iqg_ref_A"
  Bus Creator/1 -> DadosCtrlTensao/1
  Ganhos1/1(u) -> Rate Transition2/1  "igq*"
  Subsystem1/2(CE) -> Scope5/2  "CE"
  Subsystem1/1(E.) -> Scope5/1  "E"
  Gain/1 -> Ganhos1/1(E), Subsystem1/1(E)
  Discrete-Time Integrator/1 -> Scope5/3, [iqg_ref], igq*/1
  Rate Transition2/1 -> Discrete-Time Integrator/1

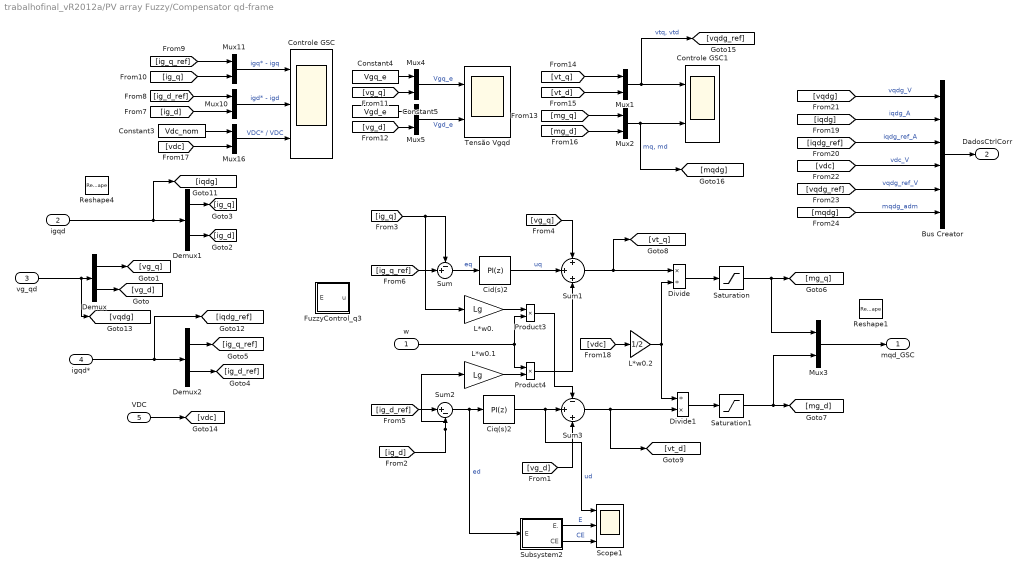
== system trabalhofinal_vR2012a/PV array Fuzzy/Compensator qd-frame ==
  w : Inport
  igqd : Inport  Port=2
  vg_qd : Inport  Port=3
  igqd* : Inport  Port=4
  VDC : Inport  Port=5
  Bus Creator : BusCreator  Inputs=6
  Cid(s)2 : simulink/Continuous/PID Controller  Controller=PI  TimeDomain=Discrete-time  SampleTime=-1  IntegratorMethod=Trapezoidal  FilterMethod=Forward Euler  Form=Parallel  UseFilter=on  ControllerParametersSource=internal  P=GSC_Ci_kp  I=GSC_Ci_ki  D=0  N=100  InitialConditionSource=internal  InitialConditionForIntegrator=GSC_Uq_e  InitialConditionForFilter=0  ExternalReset=none  LimitOutput=off  UpperSaturationLimit=inf  LowerSaturationLimit=-inf  LinearizeAsGain=on  AntiWindupMode=none  Kb=1  TrackingMode=off  Kt=1  PParamMin=[]  PParamMax=[]  IParamMin=[]  IParamMax=[]  DParamMin=[]  DParamMax=[]  NParamMin=[]  NParamMax=[]  KbParamMin=[]  KbParamMax=[]  KtParamMin=[]  KtParamMax=[]  POutMin=[]  POutMax=[]  IOutMin=[]  IOutMax=[]  DOutMin=[]  DOutMax=[]  NOutMin=[]  NOutMax=[]  KbOutMin=[]  KbOutMax=[]  KtOutMin=[]  KtOutMax=[]  IntegratorOutMin=[]  IntegratorOutMax=[]  FilterOutMin=[]  FilterOutMax=[]  SumOutMin=[]  SumOutMax=[]  SumI1OutMin=[]  SumI1OutMax=[]  SumI2OutMin=[]  SumI2OutMax=[]  SumI3OutMin=[]  SumI3OutMax=[]  SumDOutMin=[]  SumDOutMax=[]  SaturationOutMin=[]  SaturationOutMax=[]  IntegratorContinuousStateAttributes=''  IntegratorStateMustResolveToSignalObject=off  IntegratorRTWStateStorageClass=Auto  FilterContinuousStateAttributes=''  FilterStateMustResolveToSignalObject=off  FilterRTWStateStorageClass=Auto  DifferentiatorICPrevScaledInput=0  DifferentiatorOutMin=[]  DifferentiatorOutMax=[]
  Ciq(s)2 : simulink/Continuous/PID Controller  Controller=PI  TimeDomain=Discrete-time  SampleTime=-1  IntegratorMethod=Trapezoidal  FilterMethod=Forward Euler  Form=Parallel  UseFilter=on  ControllerParametersSource=internal  P=GSC_Ci_kp  I=GSC_Ci_ki  D=0  N=100  InitialConditionSource=internal  InitialConditionForIntegrator=GSC_Ud_e  InitialConditionForFilter=0  ExternalReset=none  LimitOutput=off  UpperSaturationLimit=inf  LowerSaturationLimit=-inf  LinearizeAsGain=on  AntiWindupMode=none  Kb=1  TrackingMode=off  Kt=1  PParamMin=[]  PParamMax=[]  IParamMin=[]  IParamMax=[]  DParamMin=[]  DParamMax=[]  NParamMin=[]  NParamMax=[]  KbParamMin=[]  KbParamMax=[]  KtParamMin=[]  KtParamMax=[]  POutMin=[]  POutMax=[]  IOutMin=[]  IOutMax=[]  DOutMin=[]  DOutMax=[]  NOutMin=[]  NOutMax=[]  KbOutMin=[]  KbOutMax=[]  KtOutMin=[]  KtOutMax=[]  IntegratorOutMin=[]  IntegratorOutMax=[]  FilterOutMin=[]  FilterOutMax=[]  SumOutMin=[]  SumOutMax=[]  SumI1OutMin=[]  SumI1OutMax=[]  SumI2OutMin=[]  SumI2OutMax=[]  SumI3OutMin=[]  SumI3OutMax=[]  SumDOutMin=[]  SumDOutMax=[]  SaturationOutMin=[]  SaturationOutMax=[]  IntegratorContinuousStateAttributes=''  IntegratorStateMustResolveToSignalObject=off  IntegratorRTWStateStorageClass=Auto  FilterContinuousStateAttributes=''  FilterStateMustResolveToSignalObject=off  FilterRTWStateStorageClass=Auto  DifferentiatorICPrevScaledInput=0  DifferentiatorOutMin=[]  DifferentiatorOutMax=[]
  Constant3 : Constant  Value=Vdc_nom
  Constant4 : Constant  Value=Vgq_e
  Constant5 : Constant  Value=Vgd_e
  Controle GSC : Scope  NumInputPorts=3
      settings: TimeRange=0.1  MaxDataPoints=5000  SaveToWorkspace=off  SaveName=ScopeData3  YMin=-202.56389~-13.99201~696.10446  YMax=776.93563~91.14005~1761.62108  SampleTime=-1
  Controle GSC1 : Scope  NumInputPorts=2
      settings: TimeRange=auto  MaxDataPoints=5000  SaveToWorkspace=off  SaveName=ScopeData4  YMin=-200.65446~-0.29006  YMax=720.49949~1.00993  SampleTime=-1
  Demux : Demux  Outputs=2
  Demux1 : Demux  Outputs=2
  Demux2 : Demux  Outputs=2
  Divide : Product  Inputs=*/
  Divide1 : Product  Inputs=/*
  FuzzyControl_q3 : Subsystem  mask{GE=1/(3*70), GCE=1/(7*4e4), GY=30*7}
      mask prompts: GE "Fator erro"; GCE "Fator mudança erro"; GY "Fator Saída"
  L*w0. : Gain  Gain=Lg
  L*w0.1 : Gain  Gain=Lg
  L*w0.2 : Gain  Gain=1/2
  Mux{1..5,10..11,16} (8 alike) : Mux  Inputs=2
  Product3 : Product
  Product4 : Product
  Reshape1 : Reshape  OutputDimensionality=Customize  OutputDimensions=[2,1]
  Reshape4 : Reshape  OutputDimensionality=Customize  OutputDimensions=[2,1]
  Saturation : Saturate  UpperLimit=1  LowerLimit=-1
  Saturation1 : Saturate  UpperLimit=1  LowerLimit=-1
  Scope1 : Scope  NumInputPorts=3
      settings: TimeRange=auto  MaxDataPoints=5000  SaveToWorkspace=off  SaveName=ScopeData3  YMin=-24.21242~-70.64171~-135065.73023  YMax=2.6976~24.24875~41210.34485  SampleTime=-1
  Subsystem2 : Subsystem
  Sum : Sum  Inputs=-+|
  Sum1 : Sum  Inputs=+|+|+
  Sum2 : Sum  Inputs=|+-
  Sum3 : Sum  Inputs=-|+|+
  Tensão Vgqd : Scope  NumInputPorts=2
      settings: TimeRange=auto  MaxDataPoints=5000  SaveToWorkspace=off  SaveName=ScopeData36  YMin=148.66619~-14.34464  YMax=209.64626~12.14165  SampleTime=-1
  mqd_GSC : Outport
  DadosCtrlCorr : Outport  Port=2
  wires:
  Demux/2 -> [vg_d]
  Demux/1 -> [vg_q]
  Demux1/2 -> [ig_d]
  Demux1/1 -> [ig_q]
  L*w0.2/1 -> Divide/2, Divide1/1
  [mg_q] -> Mux2/1
  [mg_d] -> Mux2/2
  [vt_q] -> Mux1/1
  [vt_d] -> Mux1/2
  Mux2/1 -> [mqdg], Controle GSC1/2  "mq, md"
  Mux1/1 -> [vqdg_ref], Controle GSC1/1  "vtq, vtd"
  [ig_q] -> Mux11/2
  [ig_q_ref] -> Mux11/1
  [ig_d] -> Mux10/2
  [ig_d_ref] -> Mux10/1
  Mux11/1 -> Controle GSC/1  "igq* - igq"
  Mux10/1 -> Controle GSC/2  "igd* - igd"
  Divide/1 -> Saturation/1
  L*w0.1/1 -> Product4/2
  [ig_q_ref] -> Sum/2
  igqd*/1 -> Demux2/1, [iqdg_ref]
  VDC/1 -> [vdc]
  Sum/1 -> Cid(s)2/1  "eq"
  [ig_d] -> L*w0.1/1, Sum2/2
  Sum1/1 -> Divide/1, [vt_q]
  Cid(s)2/1 -> Sum1/2  "uq"
  Ciq(s)2/1 -> Scope1/1, Sum3/2  "ud"
  Sum2/1 -> Ciq(s)2/1, Subsystem2/1(E)  "ed"
  Sum3/1 -> Divide1/2, [vt_d]
  L*w0./1 -> Product3/1
  [ig_d_ref] -> Sum2/1
  Mux16/1 -> Controle GSC/3  "VDC* / VDC"
  Constant3/1 -> Mux16/1
  [vdc] -> Mux16/2
  Demux2/1 -> [ig_q_ref]
  Demux2/2 -> [ig_d_ref]
  [vdc] -> L*w0.2/1
  Constant4/1 -> Mux4/1
  [vg_q] -> Mux4/2
  Constant5/1 -> Mux5/1
  [vg_d] -> Mux5/2
  Mux4/1 -> Tensão Vgqd/1  "Vgq_e"
  Mux5/1 -> Tensão Vgqd/2  "Vgd_e"
  Saturation/1 -> Mux3/1, [mg_q]
  Divide1/1 -> Saturation1/1
  Saturation1/1 -> Mux3/2, [mg_d]
  [ig_q] -> Sum/1, L*w0./1
  igqd/1 -> [iqdg], Demux1/1
  vg_qd/1 -> [vqdg], Demux/1
  Mux3/1 -> mqd_GSC/1
  [vqdg] -> Bus Creator/1  "vqdg_V"
  [iqdg] -> Bus Creator/2  "iqdg_A"
  [iqdg_ref] -> Bus Creator/3  "iqdg_ref_A"
  Bus Creator/1 -> DadosCtrlCorr/1
  [vdc] -> Bus Creator/4  "vdc_V"
  [vqdg_ref] -> Bus Creator/5  "vqdg_ref_V"
  [mqdg] -> Bus Creator/6  "mqdg_adm"
  [vg_q] -> Sum1/1
  [vg_d] -> Sum3/3
  Product3/1 -> Sum3/1
  Product4/1 -> Sum1/3
  w/1 -> Product3/2, Product4/1
  Subsystem2/2(CE) -> Scope1/3  "CE"
  Subsystem2/1(E.) -> Scope1/2  "E"

== system trabalhofinal_vR2012a/PV array Fuzzy/DSOGI1 ==
  note: Fasor = (Fq-jFd)/sqrt(2)
  angV : Inport
  V : Inport  Port=2
  I : Inport  Port=3
  Calcula Impedância2 : Subsystem
  Complex to Magnitude-Angle : ComplexToMagnitudeAngle  Output=Angle
  Complex to Magnitude-Angle1 : ComplexToMagnitudeAngle
  Fasor_Krause : Subsystem
  Fasor_Krause1 : Subsystem
  Magnitude-Angle to Complex : MagnitudeAngleToComplex
  Sum : Sum  Inputs=|++
  Terminator : Terminator
  I_fasor : Outport
  wires:
  Magnitude-Angle to Complex/1 -> I_fasor/1
  Complex to Magnitude-Angle1/2 -> Sum/1
  Complex to Magnitude-Angle1/1 -> Magnitude-Angle to Complex/1
  Complex to Magnitude-Angle/1 -> Terminator/1
  V/1 -> Calcula Impedância2/1(Vinf_abc)
  I/1 -> Calcula Impedância2/2(I_abc)
  Calcula Impedância2/1(Vinf_q) -> Fasor_Krause/1(Fq)
  Calcula Impedância2/2(Vinf_d) -> Fasor_Krause/2(Fd)
  Fasor_Krause/1(Fasor) -> Complex to Magnitude-Angle/1
  Calcula Impedância2/3(Ipac_q) -> Fasor_Krause1/1(Fq)
  Calcula Impedância2/4(Ipac_d) -> Fasor_Krause1/2(Fd)
  Fasor_Krause1/1(Fasor) -> Complex to Magnitude-Angle1/1
  Sum/1 -> Magnitude-Angle to Complex/2
  angV/1 -> Sum/2

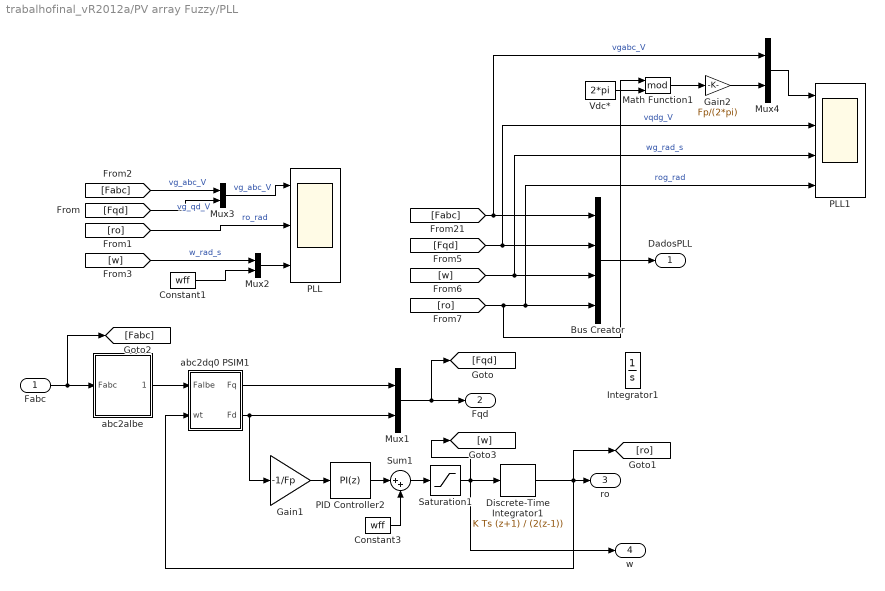
== system trabalhofinal_vR2012a/PV array Fuzzy/PLL ==
  Fabc : Inport
  Bus Creator : BusCreator  Inputs=4
  Constant1 : Constant  Value=wff
  Constant3 : Constant  Value=wff
  Discrete-Time Integrator1 : DiscreteIntegrator  IntegratorMethod=Integration: Trapezoidal  InitialCondition=ro0  InitialConditionMode=State only (most efficient)  SampleTime=-1  ICPrevOutput=DiscIntNeverNeededParam  ICPrevScaledInput=DiscIntNeverNeededParam
  Gain1 : Gain  Gain=-1/Fp
  Gain2 : Gain  Gain=Fp/(2*pi)
  Integrator1 : Integrator  InitialCondition=ro0  UpperSaturationLimit=2*pi  LowerSaturationLimit=0
  Math Function1 : Math  Operator=mod  SaturateOnIntegerOverflow=on
  Mux{1..4} (4 alike) : Mux  Inputs=2
  PID Controller2 : simulink/Continuous/PID Controller  Controller=PI  TimeDomain=Discrete-time  SampleTime=-1  IntegratorMethod=Trapezoidal  FilterMethod=Forward Euler  Form=Parallel  UseFilter=on  ControllerParametersSource=internal  P=kp  I=ki  D=1  N=100  InitialConditionSource=internal  InitialConditionForIntegrator=dw0  InitialConditionForFilter=0  ExternalReset=none  LimitOutput=off  UpperSaturationLimit=inf  LowerSaturationLimit=-inf  LinearizeAsGain=on  AntiWindupMode=none  Kb=1  TrackingMode=off  Kt=1  PParamMin=[]  PParamMax=[]  IParamMin=[]  IParamMax=[]  DParamMin=[]  DParamMax=[]  NParamMin=[]  NParamMax=[]  KbParamMin=[]  KbParamMax=[]  KtParamMin=[]  KtParamMax=[]  POutMin=[]  POutMax=[]  IOutMin=[]  IOutMax=[]  DOutMin=[]  DOutMax=[]  NOutMin=[]  NOutMax=[]  KbOutMin=[]  KbOutMax=[]  KtOutMin=[]  KtOutMax=[]  IntegratorOutMin=[]  IntegratorOutMax=[]  FilterOutMin=[]  FilterOutMax=[]  SumOutMin=[]  SumOutMax=[]  SumI1OutMin=[]  SumI1OutMax=[]  SumI2OutMin=[]  SumI2OutMax=[]  SumI3OutMin=[]  SumI3OutMax=[]  SumDOutMin=[]  SumDOutMax=[]  SaturationOutMin=[]  SaturationOutMax=[]  IntegratorContinuousStateAttributes=''  IntegratorStateMustResolveToSignalObject=off  IntegratorRTWStateStorageClass=Auto  FilterContinuousStateAttributes=''  FilterStateMustResolveToSignalObject=off  FilterRTWStateStorageClass=Auto  DifferentiatorICPrevScaledInput=0  DifferentiatorOutMin=[]  DifferentiatorOutMax=[]
  PLL : Scope  NumInputPorts=3
      settings: TimeRange=auto  MaxDataPoints=5000  SaveToWorkspace=off  SaveName=ScopeData  YMin=-224.53656~-6.47953~126.78086  YMax=224.53656~42.60785~2394.62118  SampleTime=-1
  PLL1 : Scope  NumInputPorts=4
      settings: TimeRange=auto  MaxDataPoints=5000  SaveToWorkspace=off  SaveName=ScopeData2  YMin=-269.40768~-38.60155~255.14783~-8.61315  YMax=269.40768~230.45378~521.85676~62.01096  SampleTime=-1
  Saturation1 : Saturate  UpperLimit=10*wff  LowerLimit=-0.1*wff
  Sum1 : Sum  Inputs=|++
  Vdc* : Constant  Value=2*pi  SampleTime=-1
  abc2albe : Subsystem
  abc2dq0 PSIM1 : Subsystem
  DadosPLL : Outport
  Fqd : Outport  Port=2
  ro : Outport  Port=3
  w : Outport  Port=4
  wires:
  abc2albe/1(Falbe) -> abc2dq0 PSIM1/1(Falbe)
  abc2dq0 PSIM1/2(Fd) -> Gain1/1, Mux1/2
  Constant3/1 -> Sum1/2
  abc2dq0 PSIM1/1(Fq) -> Mux1/1
  Sum1/1 -> Saturation1/1
  Gain1/1 -> PID Controller2/1
  PID Controller2/1 -> Sum1/1
  Mux3/1 -> PLL/1  "vg_abc_V"
  Fabc/1 -> abc2albe/1(Fabc), [Fabc]
  [ro] -> PLL/2  "ro_rad"
  [Fqd] -> Mux3/2  "vg_qd_V"
  Mux1/1 -> Fqd/1, [Fqd]
  [w] -> Mux2/1  "w_rad_s"
  Mux2/1 -> PLL/3
  Constant1/1 -> Mux2/2
  [Fabc] -> Mux4/1, Bus Creator/1  "vgabc_V"
  [Fqd] -> PLL1/2, Bus Creator/2  "vqdg_V"
  [w] -> PLL1/3, Bus Creator/3  "wg_rad_s"
  Bus Creator/1 -> DadosPLL/1
  [ro] -> Math Function1/1, PLL1/4, Bus Creator/4  "rog_rad"
  [Fabc] -> Mux3/1  "vg_abc_V"
  Saturation1/1 -> w/1, Discrete-Time Integrator1/1, [w]
  Discrete-Time Integrator1/1 -> [ro], abc2dq0 PSIM1/2(wt), ro/1
  Vdc*/1 -> Math Function1/2
  Math Function1/1 -> Gain2/1
  Mux4/1 -> PLL1/1
  Gain2/1 -> Mux4/2

== system trabalhofinal_vR2012a/PV array Fuzzy/PWM ==
  mabc : Inport
  PWM Generator1 : powerlib_extras/Control  Blocks/PWM Generator  GeneratorMode="3-arm  bridge (6 pulses)"  Fc=PWM_freq_grid  Internal=off  mIndex=0.4  Freq=60  Phase=0
  Unit Delay4 : UnitDelay  SampleTime=-1
  Pulses : Outport
  wires:
  PWM Generator1/1 -> Pulses/1
  mabc/1 -> PWM Generator1/1

== system trabalhofinal_vR2012a/PV array Fuzzy/Subsystem ==
  Current Measurement : powerlib/Measurements/Current Measurement  PhasorSimulation=off  OutputType=Complex  PSBequivalent=0
  vbn : powerlib/Measurements/Voltage Measurement  PhasorSimulation=off  OutputType=Complex  PSBequivalent=0
  A : PMIOPort  Port=1  Side=Left
  a : PMIOPort  Port=2  Side=Right
  B : PMIOPort  Port=3  Side=Left
  Vdc : Outport
  Idc : Outport  Port=2
  wires:
  Current Measurement/1 -> Idc/1
  vbn/1 -> Vdc/1
  connections:
  Current Measurement/LConn1 -- a/RConn1
  vbn/LConn2 -- B/RConn1
  vbn/LConn1 -- A/RConn1 -- Current Measurement/RConn1

== system trabalhofinal_vR2012a/PV array Fuzzy/abc2dq0 PSIM1 ==
  Fabc : Inport
  wt : Inport  Port=2
  Mux1 : Mux  Inputs=2
  abc2albe : Subsystem
  abc2dq0 PSIM1 : Subsystem
  Fqd : Outport
  wires:
  abc2albe/1(Falbe) -> abc2dq0 PSIM1/1(Falbe)
  abc2dq0 PSIM1/2(Fd) -> Mux1/2
  abc2dq0 PSIM1/1(Fq) -> Mux1/1
  Mux1/1 -> Fqd/1
  wt/1 -> abc2dq0 PSIM1/2(wt)
  Fabc/1 -> abc2albe/1(Fabc)

== system trabalhofinal_vR2012a/PV array Fuzzy/dq02abc PSIM ==
  Fqd : Inport
  wt : Inport  Port=2
  abc2dq0 PSIM : Subsystem
  albe2abc : Subsystem
  Fabc : Outport
  wires:
  albe2abc/1(Fabc) -> Fabc/1
  abc2dq0 PSIM/1(Falbe) -> albe2abc/1(Falbe)
  wt/1 -> abc2dq0 PSIM/2(wt)
  Fqd/1 -> abc2dq0 PSIM/1(Fqd)
